simulink model "PID_controller_MC"  (R2020a)
settings: Solver=VariableStepAuto  StartTime=0.0  StopTime=10.0  RelTol=1e-3
model mask{Kd=0, Ki=0, Kp=0}
  mask prompts: Kd "Derivative Gain    [Kd]"; Ki "Integral Gain        [Ki]"; Kp "Proportional Gain [Kp]"
model workspace (MAT data in the model file):
  Kd = 0
  Ki = 0
  Kp = 0
settings Model: DataDictionary=DataDictionaryMotorPositionControlPID.sldd  ParameterArgumentNames=Kd,Ki,Kp  Creator=DELL  LastModifiedBy=DELL
settings DataIOCC: SaveOutput=off  SaveTime=off

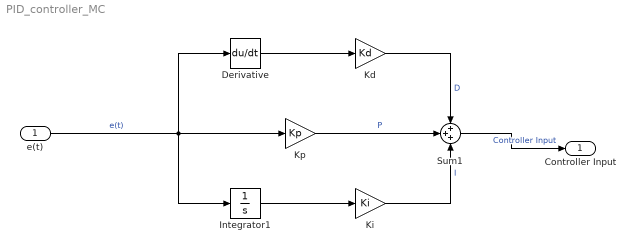
== system PID_controller_MC ==
  e(t) : Inport  OutDataTypeStr=double  PortDimensions=1  SampleTime=0
  Derivative : Derivative
  Integrator1 : Integrator
  Kd : Gain  Gain=Kd
  Ki : Gain  Gain=Ki
  Kp : Gain  Gain=Kp
  Sum1 : Sum  Inputs=+++
  Controller Input : Outport  OutDataTypeStr=double  PortDimensions=1  SampleTime=0
  wires:
  Ki/1 -> Sum1/3  "I"
  Derivative/1 -> Kd/1
  e(t)/1 -> Derivative/1, Kp/1, Integrator1/1  "e(t)"
  Integrator1/1 -> Ki/1
  Kd/1 -> Sum1/1  "D"
  Sum1/1 -> Controller Input/1  "Controller Input"
  Kp/1 -> Sum1/2  "P"
